simulink model "testuart"  (R2013a)
settings: Solver=FixedStepDiscrete  StartTime=0.0  StopTime=inf  FixedStep=0.001  RelTol=1e-3
undefined symbols (not defined in the file or in its folder): LF, serial
libraries: simulink x2, instrumentlib x2
settings Model: Creator=User  LastModifiedBy=User
settings DataIOCC: LimitDataPoints=off

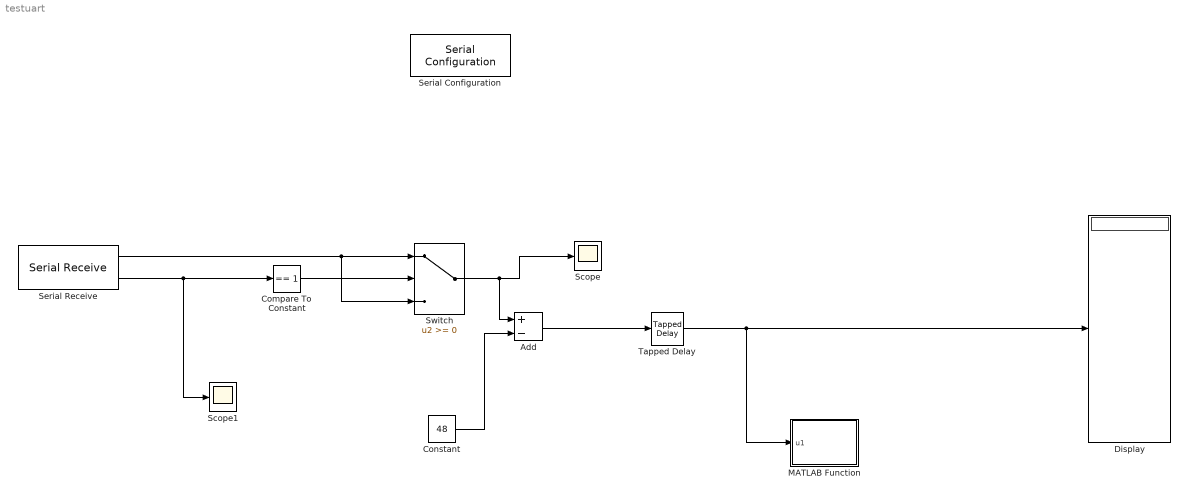
== system testuart ==
  Add : Sum  Inputs=+-
  Compare To Constant : simulink/Logic and Bit Operations/Compare To Constant  relop===  const=1  OutDataTypeStr=boolean
  Constant : Constant  Value=48
  Display : Display
  MATLAB Function : MATLAB Function  TreatAsAtomicUnit=on
  Scope : Scope
      settings: YMin=10  YMax=60
  Scope1 : Scope
      settings: YMin=1  YMax=1
  Serial Configuration : instrumentlib/Serial Configuration  Priority=-200000  ComPortMenu=COM7  ComPort=COM7  ObjConstructor=serial('COM7');  BaudRate=57600  DataBits=8  Parity=none  StopBits=1  FlowControl=none  Timeout=10  ByteOrder=LittleEndian
  Serial Receive : instrumentlib/Serial Receive  ComPortMenu=COM7  ComPort=COM7  ObjConstructor=serial('COM7');  Terminator=LF ('\n')  DataSize=[1 1]  DataType=uint8  EnableBlockingMode=off  ActionDataUnavailable=Output custom value  CustomValue=0  SampleTime=0.001
  Switch : Switch
  Tapped Delay : simulink/Discrete/Tapped Delay  vinit=0.0  samptime=-1  NumDelays=10  DelayOrder=Oldest  includeCurrent=off
  wires:
  Tapped Delay/1 -> MATLAB Function/1(u1), Display/1
  Add/1 -> Tapped Delay/1
  Constant/1 -> Add/2
  Serial Receive/2 -> Scope1/1, Compare To Constant/1
  Compare To Constant/1 -> Switch/2
  Serial Receive/1 -> Switch/3, Switch/1
  Switch/1 -> Add/1, Scope/1

== matlab function testuart/MATLAB Function ==
  data: u1 input
function fcn(u1)

plot(u1);

end
